simulink model "matrix6_1"  (R2020a)
settings: Solver=VariableStepAuto  StartTime=0.0  StopTime=1  RelTol=1e-6
model workspace (MAT data in the model file):
  A1 = 0.212
  A2 = 0.0033
  B1 = 0.311
  B2 = 0.0075
  C1 = 0.1
  C2 = 0.0084
  Ce1 = 0.27
  Ce2 = 0.12
  Cm1 = 0.36
  Cm2 = 0.12
  D1 = 0.1
  D2 = 0.001
  E1 = 0.1
  E2 = 0.001
  F1 = 0.1
  F2 = 0.001
  L1 = 0.00032
  L2 = 0.000194
  R1 = 0.32
  R2 = 0.485
  Xc2 = 0
  Yc2 = 0.0148
  dt1 = 0.6
  dt2 = 0.6
  dx1 = 3.14
  dx2 = 1.57
  g = 9.81
  m2 = 1.13085
(part 2 of 2)

== system matrix6_1/Object/W(t,q)/w beta (t, q)/bracket2/Subsystem/D(beta)2 ==
  beta : Inport
  Gain : Gain  Gain=D2
  Gain2 : Gain  Gain=E2
  Sum : Sum
  Trigonometric Function : Trigonometry  Operator=cos
  Trigonometric Function2 : Trigonometry
  D : Outport  VectorParamsAs1DForOutWhenUnconnected=off
  wires:
  Trigonometric Function/1 -> Gain/1
  Trigonometric Function2/1 -> Gain2/1
  beta/1 -> Trigonometric Function2/1, Trigonometric Function/1
  Gain/1 -> Sum/1
  Sum/1 -> D/1
  Gain2/1 -> Sum/2

== system matrix6_1/Object/W(t,q)/w beta (t, q)/bracket2/Subsystem/F(beta) ==
  beta : Inport
  Gain : Gain  Gain=F2
  Gain1 : Gain  Gain=2
  Gain2 : Gain  Gain=(A2-B2)/2
  Sum : Sum  Inputs=+-
  Trigonometric Function : Trigonometry  Operator=cos
  Trigonometric Function2 : Trigonometry
  F : Outport  VectorParamsAs1DForOutWhenUnconnected=off
  wires:
  Gain1/1 -> Trigonometric Function2/1
  Gain2/1 -> Sum/2
  Sum/1 -> F/1
  Gain/1 -> Sum/1
  beta/1 -> Gain1/1, Trigonometric Function/1
  Trigonometric Function2/1 -> Gain2/1
  Trigonometric Function/1 -> Gain/1

== system matrix6_1/Object/W(t,q)/w beta (t, q)/bracket2/Subsystem/F(beta)1 ==
  beta : Inport
  Gain : Gain  Gain=F2
  Gain1 : Gain  Gain=2
  Gain2 : Gain  Gain=(A2-B2)/2
  Sum : Sum  Inputs=+-
  Trigonometric Function : Trigonometry  Operator=cos
  Trigonometric Function2 : Trigonometry
  F : Outport  VectorParamsAs1DForOutWhenUnconnected=off
  wires:
  Trigonometric Function/1 -> Gain/1
  Trigonometric Function2/1 -> Gain2/1
  beta/1 -> Trigonometric Function/1, Gain1/1
  Gain/1 -> Sum/1
  Sum/1 -> F/1
  Gain2/1 -> Sum/2
  Gain1/1 -> Trigonometric Function2/1

== system matrix6_1/Object/W(t,q)/w beta (t, q)/bracket2/Subsystem/F(beta)2 ==
  beta : Inport
  Gain : Gain  Gain=F2
  Gain1 : Gain  Gain=2
  Gain2 : Gain  Gain=(A2-B2)/2
  Sum : Sum  Inputs=+-
  Trigonometric Function : Trigonometry  Operator=cos
  Trigonometric Function2 : Trigonometry
  F : Outport  VectorParamsAs1DForOutWhenUnconnected=off
  wires:
  Trigonometric Function/1 -> Gain/1
  Trigonometric Function2/1 -> Gain2/1
  beta/1 -> Trigonometric Function/1, Gain1/1
  Gain/1 -> Sum/1
  Sum/1 -> F/1
  Gain2/1 -> Sum/2
  Gain1/1 -> Trigonometric Function2/1

== system matrix6_1/Object/W(t,q)/w beta (t, q)/bracket2/Subsystem1/A2(beta) ==
  beta : Inport
  Gain : Gain  Gain=A2-B2
  Gain1 : Gain  Gain=2
  Gain2 : Gain  Gain=F2
  Gain3 : Gain  Gain=1/2
  Sum : Sum
  Trigonometric Function : Trigonometry  Operator=cos
  Trigonometric Function2 : Trigonometry
  A2 : Outport  VectorParamsAs1DForOutWhenUnconnected=off
  wires:
  Trigonometric Function/1 -> Gain/1
  Trigonometric Function2/1 -> Gain2/1
  beta/1 -> Gain1/1
  Gain/1 -> Gain3/1
  Sum/1 -> A2/1
  Gain2/1 -> Sum/2
  Gain1/1 -> Trigonometric Function/1, Trigonometric Function2/1
  Gain3/1 -> Sum/1

== system matrix6_1/Object/W(t,q)/w beta (t, q)/bracket2/Subsystem1/E(beta) ==
  beta : Inport
  Gain : Gain  Gain=E2
  Gain2 : Gain  Gain=D2
  Sum : Sum  Inputs=+-
  Trigonometric Function : Trigonometry  Operator=cos
  Trigonometric Function2 : Trigonometry
  E : Outport  VectorParamsAs1DForOutWhenUnconnected=off
  wires:
  Gain2/1 -> Sum/2
  Sum/1 -> E/1
  Gain/1 -> Sum/1
  beta/1 -> Trigonometric Function/1, Trigonometric Function2/1
  Trigonometric Function2/1 -> Gain2/1
  Trigonometric Function/1 -> Gain/1

== system matrix6_1/Object/W(t,q)/w beta (t, q)/bracket2/Subsystem2/D(beta) ==
  beta : Inport
  Gain : Gain  Gain=D2
  Gain2 : Gain  Gain=E2
  Sum : Sum
  Trigonometric Function : Trigonometry  Operator=cos
  Trigonometric Function2 : Trigonometry
  D : Outport  VectorParamsAs1DForOutWhenUnconnected=off
  wires:
  Gain2/1 -> Sum/2
  Sum/1 -> D/1
  Gain/1 -> Sum/1
  beta/1 -> Trigonometric Function/1, Trigonometric Function2/1
  Trigonometric Function2/1 -> Gain2/1
  Trigonometric Function/1 -> Gain/1

== system matrix6_1/Object/W(t,q)/w beta (t, q)/bracket2/Subsystem2/F(beta) ==
  beta : Inport
  Gain : Gain  Gain=F2
  Gain1 : Gain  Gain=2
  Gain2 : Gain  Gain=(A2-B2)/2
  Sum : Sum  Inputs=+-
  Trigonometric Function : Trigonometry  Operator=cos
  Trigonometric Function2 : Trigonometry
  F : Outport  VectorParamsAs1DForOutWhenUnconnected=off
  wires:
  Trigonometric Function/1 -> Gain/1
  Trigonometric Function2/1 -> Gain2/1
  beta/1 -> Trigonometric Function/1, Gain1/1
  Gain/1 -> Sum/1
  Sum/1 -> F/1
  Gain2/1 -> Sum/2
  Gain1/1 -> Trigonometric Function2/1

== system matrix6_1/Object/W(t,q)/w beta (t, q)/bracket2/Subsystem3/A2(beta) ==
  beta : Inport
  Gain : Gain  Gain=A2-B2
  Gain1 : Gain  Gain=2
  Gain2 : Gain  Gain=F2
  Gain3 : Gain  Gain=1/2
  Sum : Sum
  Trigonometric Function : Trigonometry  Operator=cos
  Trigonometric Function2 : Trigonometry
  A2 : Outport  VectorParamsAs1DForOutWhenUnconnected=off
  wires:
  Gain3/1 -> Sum/1
  Gain1/1 -> Trigonometric Function2/1, Trigonometric Function/1
  Gain2/1 -> Sum/2
  Sum/1 -> A2/1
  Gain/1 -> Gain3/1
  beta/1 -> Gain1/1
  Trigonometric Function2/1 -> Gain2/1
  Trigonometric Function/1 -> Gain/1

== system matrix6_1/Object/W(t,q)/w beta (t, q)/bracket2/Subsystem3/E(beta) ==
  beta : Inport
  Gain : Gain  Gain=E2
  Gain2 : Gain  Gain=D2
  Sum : Sum  Inputs=+-
  Trigonometric Function : Trigonometry  Operator=cos
  Trigonometric Function2 : Trigonometry
  E : Outport  VectorParamsAs1DForOutWhenUnconnected=off
  wires:
  Trigonometric Function/1 -> Gain/1
  Trigonometric Function2/1 -> Gain2/1
  beta/1 -> Trigonometric Function2/1, Trigonometric Function/1
  Gain/1 -> Sum/1
  Sum/1 -> E/1
  Gain2/1 -> Sum/2
